simulink model "lookForPath_mod"  (Simulink 7.6)
settings: Solver=FixedStepDiscrete  StartTime=0.0  StopTime=0  RelTol=1e-3
values from neighbouring files (symbols this model uses):
  Track_HueHigher = .1    (= 0.1)    [VisionConstants.m]
  Track_HueLower = .25    (= 0.25)    [VisionConstants.m]
  Track_Min_Eccentricity = 0.9    [VisionConstants.m]
  Track_Saturation = 0.5    [VisionConstants.m]
undefined symbols (not defined in the file or in its folder): Rec, SDTV
libraries: simulink x3, vipstatistics x1, vipconversions x1, viptextngfix x1
settings Model: Creator=auvt  LastModifiedBy=Administrator  RecordCoverage=on  CovHTMLOptions=-aTS=1 -bRG=1 -bTC=1 -hTR=0 -nFC=0 -scm=1 -bcm=1 -xEv=0  CovModelRefEnable=all  CovExternalEMLEnable=on

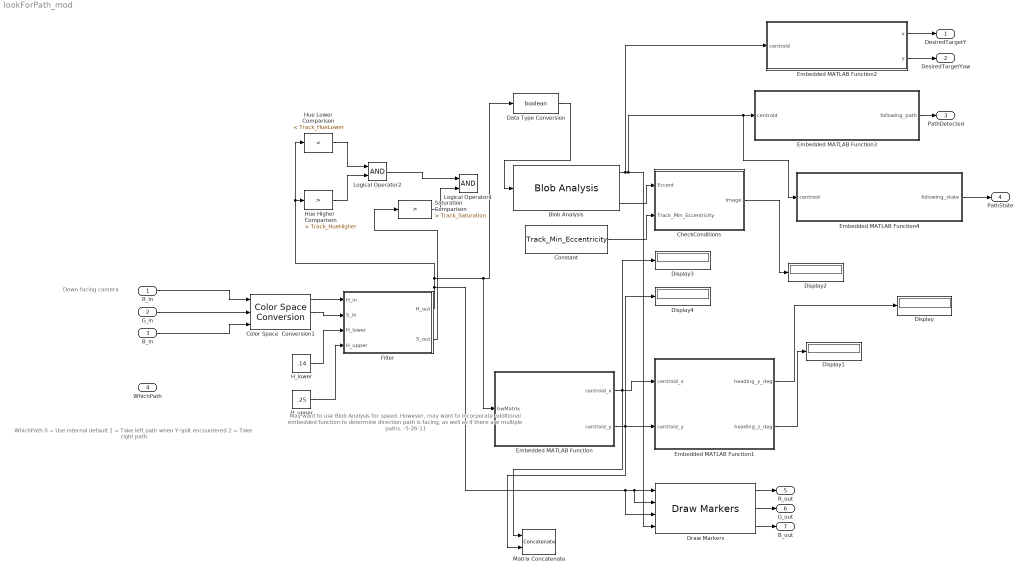
== system lookForPath_mod ==
  note: May want to use Blob Analysis for speed.
      | However, may want to incorporate
      | additional embedded function to
      | determine direction path is facing,
      | as well as if there are multiple paths.
      |
      | -5-26-11
  note: Down-facing camera
  note: WhichPath
      | 0 = Use internal default
      | 1 = Take left path when Y-split encountered
      | 2 = Take right path
  R_in : Inport  PortDimensions=[120 160]
  G_in : Inport  Port=2  PortDimensions=[120 160]
  B_in : Inport  Port=3  PortDimensions=[120 160]
  WhichPath : Inport  Port=4
  Blob Analysis : vipstatistics/Blob Analysis  Tag=vipblks_row_conv  DialogController=vipDDGCreate  DialogControllerArgs=DataTag0  area=off  centroid=on  bBox=on  majorAxis=off  minorAxis=off  angle=off  eccentricity=on  equivDiameterSq=off  extent=off  perimeter=off  maxBlobs=Max_Num_Blobs  warnIfNumBlobsExceeded=on  isCount=off  useMinArea=on  minArea=Min_Blob_Size  useMaxArea=on  maxArea=Max_Blob_Size  excludeBorderBlob=off  outDT=double  isOutVarDim=off  isFill=on  fillValues=-1  conn=8  isLabel=off  outputMode=Binary point scaling  outputWordLength=32  outputFracLength=16  firstCoeffMode=Binary point scaling  firstCoeffWordLength=16  firstCoeffFracLength=14  secondCoeffMode=Binary point scaling  secondCoeffWordLength=32  secondCoeffFracLength=16  accumMode=Binary point scaling  accumWordLength=32  accumFracLength=0  prodOutputMode=Binary point scaling  prodOutputWordLength=32  prodOutputFracLength=16  roundingMode=Floor  overflowMode=off
  CheckConditions : Stateflow chart  TreatAsAtomicUnit=on
  Color Space  Conversion1 : vipconversions/Color Space  Conversion  conversion=Obsolete  conversionActive=R'G'B' to HSV  wp_str=D65  rec=Rec. 601 (SDTV)  sys=1125/60/2:1  imagePorts=Separate color signals
  Constant : Constant  Value=Track_Min_Eccentricity  SampleTime=-1
  Data Type Conversion : DataTypeConversion  OutDataTypeStr=boolean
  Display{,1..4} (5 alike) : Display
  Draw Markers : viptextngfix/Draw Markers  DialogController=vipDDGCreate  DialogControllerArgs=DataTag1  shape=X-mark  size=7  fill=off  fillClrSource=Specify via dialog  display=User-specified value  intensity=200  color=[0 1 0]  opacity=0.6  viewport=Entire image  antialiasing=off  inType=Obsolete  imagePorts=Separate color signals  prodOutputMode=Binary point scaling  prodOutputWordLength=32  prodOutputFracLength=14  memoryMode=Specify word length  memoryWordLength=16  memoryFracLength=15  roundingMode=Floor  overflowMode=off
  Embedded MATLAB Function : Stateflow chart  TreatAsAtomicUnit=on
  Embedded MATLAB Function1 : Stateflow chart  TreatAsAtomicUnit=on
  Embedded MATLAB Function2 : Stateflow chart  TreatAsAtomicUnit=on
  Embedded MATLAB Function3 : Stateflow chart  TreatAsAtomicUnit=on
  Embedded MATLAB Function4 : Stateflow chart  TreatAsAtomicUnit=on
  Filter : Stateflow chart  TreatAsAtomicUnit=on
  H_lower : Constant  Value=.14  SampleTime=-1
  H_upper : Constant  Value=.25  SampleTime=-1
  Hue Higher Comparison : simulink/Logic and Bit Operations/Compare To Constant  SystemSampleTime=-1  relop=>  const=Track_HueHigher  LogicOutDataTypeMode=boolean  ZeroCross=off
  Hue Lower Comparison : simulink/Logic and Bit Operations/Compare To Constant  SystemSampleTime=-1  relop=<  const=Track_HueLower  LogicOutDataTypeMode=boolean  ZeroCross=off
  Logical Operator1 : Logic  AllPortsSameDT=off  OutDataTypeStr=boolean
  Logical Operator2 : Logic  AllPortsSameDT=off  OutDataTypeStr=boolean
  Matrix Concatenate : Concatenate  Mode=Multidimensional array  ConcatenateDimension=2
  Saturation Comparison : simulink/Logic and Bit Operations/Compare To Constant  SystemSampleTime=-1  relop=>  const=Track_Saturation  LogicOutDataTypeMode=boolean  ZeroCross=off
  DesiredTargetY : Outport  OutDataTypeStr=double
  DesiredTargetYaw : Outport  Port=2  OutDataTypeStr=double
  PathDetected : Outport  Port=3  OutDataTypeStr=double
  PathState : Outport  Port=4  OutDataTypeStr=double
  R_out : Outport  Port=5  OutDataTypeStr=double
  G_out : Outport  Port=6  OutDataTypeStr=double
  B_out : Outport  Port=7  OutDataTypeStr=double
  wires:
  CheckConditions/1(Image) -> Display2/1
  Constant/1 -> CheckConditions/2(Track_Min_Eccentricity)
  Saturation Comparison/1 -> Logical Operator1/2
  Logical Operator2/1 -> Logical Operator1/1
  Hue Higher Comparison/1 -> Logical Operator2/2
  Hue Lower Comparison/1 -> Logical Operator2/1
  Embedded MATLAB Function/1(centroid_x) -> Embedded MATLAB Function1/1(centroid_x), Display3/1, Matrix Concatenate/1
  Embedded MATLAB Function/2(centroid_y) -> Display4/1, Embedded MATLAB Function1/2(centroid_y), Matrix Concatenate/2
  Embedded MATLAB Function1/1(heading_y_deg) -> Display/1
  Embedded MATLAB Function1/2(heading_z_deg) -> Display1/1
  Blob Analysis/3 -> CheckConditions/1(Eccent)
  Blob Analysis/1 -> Embedded MATLAB Function2/1(centroid), Draw Markers/4, Embedded MATLAB Function3/1(centroid), Embedded MATLAB Function4/1(centroid)
  Embedded MATLAB Function2/2(y) -> DesiredTargetYaw/1
  Embedded MATLAB Function2/1(x) -> DesiredTargetY/1
  Embedded MATLAB Function3/1(following_path) -> PathDetected/1
  Embedded MATLAB Function4/1(following_state) -> PathState/1
  Filter/2(S_out) -> Saturation Comparison/1
  Filter/1(H_out) -> Draw Markers/1, Draw Markers/2, Draw Markers/3, Hue Lower Comparison/1, Hue Higher Comparison/1, Embedded MATLAB Function/1(bwMatrix), Data Type Conversion/1
  Color Space  Conversion1/1 -> Filter/1(H_in)
  Color Space  Conversion1/2 -> Filter/2(S_in)
  R_in/1 -> Color Space  Conversion1/1
  B_in/1 -> Color Space  Conversion1/3
  Draw Markers/1 -> R_out/1
  G_in/1 -> Color Space  Conversion1/2
  Draw Markers/2 -> G_out/1
  Draw Markers/3 -> B_out/1
  H_lower/1 -> Filter/3(H_lower)
  H_upper/1 -> Filter/4(H_upper)
  Data Type Conversion/1 -> Blob Analysis/1

== matlab function CheckConditions ==
  data: Eccent input double; Image output double; Track_Min_Eccentricity input double
function Image = CheckConditions(Eccent, Track_Min_Eccentricity)
% This function checks the conditions to decide if a track is present

if(Eccent > Track_Min_Eccentricity)
    Image = 1;
else
    Image = 0;
end

return

== matlab function Embedded MATLAB Function ==
  data: bwMatrix input double; centroid_x output double; centroid_y output double

function [centroid_x, centroid_y] = CentroidVertScan(bwMatrix)

centroid_x = 0;
centroid_y = 0;

%{
%Author: Yama Habib
%Revision: 10/27/2010
%CentroidVertScan takes a black and white matrix (the expected output of
%the blob detection algorithm) with a single (rectangular) object detected,
%and returns the raw matrix coordinate of the centroid of the object. To
%convert to an angular heading, use the Centroid2Heading function.

%Should these be parameters? I think they're fine as constants.
WIDTH = size(bwMatrix, 2);
HEIGHT = size(bwMatrix, 1);

%increase the x step to increase efficiency. The further this
%number is from 1, the closer the object will have to be to be detected
%NOTE: find the max distance the hedge will be from the AUV, then find the
%optimal (lowest working) x step for that distance!
X_STEP = 1;
Y_STEP = 1;

%Don't detect lines unless they are longer than HEIGHT*THRESHOLD
THRESHOLD = 0.1;

%Allocate arrays...allocate more or less memory depending on how many lines
%are found in the average case
lineLengths = zeros(WIDTH,1);
lineMidpts_y = zeros(WIDTH,1);
lineMidpts_x = zeros(WIDTH,1);

%Find vertical lines
index = 1;
i = 1;
while(i <= WIDTH)
    j = 1;
    while(j <= HEIGHT)
        %skip whitespace
        while(bwMatrix(j,floor(i)) == 0)
%        while(bwMatrix(floor(i),j) == 0)
            j = j+1;
            if(j > HEIGHT)
                break;
            end
        end
        %count contiguous blackspace
        if(j <= HEIGHT)
            length = 0;
            midpt = j;
            while(bwMatrix(floor(i),j) ~= 0)
                length = length+1;
                j = j+1;
                if(j > HEIGHT)
                    break;
                end
            end
            midpt = midpt + length/2;
            %only register as a line if longer than HEIGHT*THRESHOLD
            if(length > HEIGHT*THRESHOLD)
                lineLengths(index) = length;
                lineMidpts_y(index) = midpt;
                lineMidpts_x(index) = floor(i);
                index = index+1;
            end
        end
        %rinse, repeat
    end
    i = i+X_STEP;
end

%Find maximum (longest rightmost) and minimum (longest leftmost) vertical
%lines
i = 1;
min = 1;
max = 1;
while(i <= index);
    
    % The following comparisons seek to minimize and maximize the metric
    %   " length*( width - x_midpt ) ". This effectively finds the largest
    %   leftmost and rightmost vertical lines.
    
    % This if statement should be "<" instead of ">" ??
    if(lineLengths(i)*(WIDTH-lineMidpts_x(i)) > lineLengths(min)*(WIDTH-lineMidpts_x(min)))
        min = i;
    end
    % This if statement should be correct
    if(lineLengths(i)*(lineMidpts_x(i)) >= lineLengths(max)*(lineMidpts_x(max)))
        max = i;
    end
    i = i+1;
end

%The centroid is (should be) the midpoint between the max's midpoint and
%the min's midpoint
% The assumption made is that the rightmost and leftmost lines bound a
% vertically-oriented rectangular path
centroid_x = (lineMidpts_x(min) + lineMidpts_x(max))/2;
centroid_y = (lineMidpts_y(min) + lineMidpts_y(max))/2;
end











%}










%{

% The following is the old code:







function [centroid_x, centroid_y] = CentroidVertScan(bwMatrix)
%Author: Yama Habib
%Revision: 10/27/2010
%CentroidVertScan takes a black and white matrix (the expected output of
%the blob detection algorithm) with a single (rectangular) object detected,
%and returns the raw matrix coordinate of the centroid of the object. To
%convert to an angular heading, use the Centroid2Heading function.

%Should these be parameters? I think they're fine as constants.
WIDTH = size(bwMatrix, 2);
HEIGHT = size(bwMatrix, 1);
%WIDTH = 160;
%HEIGHT = 120;

%increase the x step to increase efficiency. The further this
%number is from 1, the closer the object will have to be to be detected
%NOTE: find the max distance the hedge will be from the AUV, then find the
%optimal (lowest working) x step for that distance!
X_STEP = 1;

%Don't detect lines unless they are longer than HEIGHT*THRESHOLD
THRESHOLD = 0.1;

%Allocate arrays...allocate more or less memory depending on how many lines
%are found in the average case
lineLengths = zeros(WIDTH,1);
lineMidpts_y = zeros(WIDTH,1);
lineMidpts_x = zeros(WIDTH,1);

%Find vertical lines
index = 1;
i = 1;
while(i <= WIDTH)
    j = 1;
    while(j <= HEIGHT)
        %skip whitespace
        while(bwMatrix(j,floor(i)) == 0)
%        while(bwMatrix(floor(i),j) == 0)
            j = j+1;
            if(j > HEIGHT)
                break;
            end
        end
        %count contiguous blackspace
        if(j <= HEIGHT)
            length = 0;
            midpt = j;
            while(bwMatrix(floor(i),j) ~= 0)
                length = length+1;
                j = j+1;
                if(j > HEIGHT)
                    break;
                end
            end
            midpt = midpt + length/2;
            %only register as a line if longer than HEIGHT*THRESHOLD
            if(length > HEIGHT*THRESHOLD)
                lineLengths(index) = length;
                lineMidpts_y(index) = midpt;
                lineMidpts_x(index) = floor(i);
                index = index+1;
            end
        end
        %rinse, repeat
    end
    i = i+X_STEP;
end

%Find maximum (longest rightmost) and minimum (longest leftmost) vertical
%lines
i = 1;
min = 1;
max = 1;
while(i <= index);
    
    % The following comparisons seek to minimize and maximize the metric
    %   " length*( width - x_midpt ) ". This effectively finds the largest
    %   leftmost and rightmost vertical lines.
    
    % This if statement should be "<" instead of ">" ??
    if(lineLengths(i)*(WIDTH-lineMidpts_x(i)) > lineLengths(min)*(WIDTH-lineMidpts_x(min)))
        min = i;
    end
    % This if statement should be correct
    if(lineLengths(i)*(lineMidpts_x(i)) >= lineLengths(max)*(lineMidpts_x(max)))
        max = i;
    end
    i = i+1;
end

%The centroid is (should be) the midpoint between the max's midpoint and
%the min's midpoint
% The assumption made is that the rightmost and leftmost lines bound a
% vertically-oriented rectangular path
centroid_x = (lineMidpts_x(min) + lineMidpts_x(max))/2;
centroid_y = (lineMidpts_y(min) + lineMidpts_y(max))/2;
end

%}

== matlab function Embedded MATLAB Function1 ==
  data: centroid_x input double; heading_y_deg output double; centroid_y input double; heading_z_deg output double
function [heading_y_deg, heading_z_deg] = Centroid2Heading(centroid_x, centroid_y)
%Author: Yama Habib
%Revision: 10/27/2010
%Centroid2Heading takes a raw matrix centroid coordinate and converts
%it into a correction heading, in degrees (i.e. heading_y_deg = -30,
%heading_z_deg = 45 means that in order to orient yourself so that the
%object in question is centered in the video feed, you need to turn 30
%degrees to the left and 45 degrees upwards, assuming the camera is mounted
%on the front) The probability that this function will return exactly 0
%degrees is laughably low, so applying a reasonable threshold to the
%result is strongly recommended.

%Should these be parameters? I think they're fine as constants.
WIDTH = 160;
HEIGHT = 120;
MAXANGLE = 130;

heading_y_deg = ((centroid_x-(WIDTH/2)) / (WIDTH/2)) * (MAXANGLE/2);
heading_z_deg = ((centroid_y-(HEIGHT/2)) / (HEIGHT/2)) * (MAXANGLE/2);
end

== matlab function Embedded MATLAB Function2 ==
  data: x output double; centroid input double; y output double
function [x, y] = separate_centroids(centroid)

x = centroid(1);
y = centroid(2);

== matlab function Embedded MATLAB Function3 ==
  data: following_path output double; centroid input double
function following_path = separate_centroids(centroid)

% If at least one path element is found, then report that the path is being
% followed
if(size(centroid,1) ~= 0)
    following_path = 1;
else
    following_path = 0;
end

== matlab function Embedded MATLAB Function4 ==
  data: following_state output double; centroid input double
function following_state = separate_centroids(centroid)

% Editing note:
%   -centroid is not a useful input. This function has yet to be written.
%      -5-27-11


% Determine whether:
%   0 = No path is being followed
%   1 = A single path (can be made up of n path elements along one line)
%         is being followed
%   2 = A Y-split is being encountered
%   3 = A Y-join is being encountered

following_state = 1;

== matlab function Filter ==
  data: H_in input double; S_in input double; H_lower input double; H_upper input double; H_out output double; S_out output double
function [H_out, S_out] = path_filter(H_in, S_in, H_lower, H_upper)
% This function extracts the pixels containing hues that path elements are
%   expected to have


% Initialize
H_out = double(H_in);
S_out = double(S_in);


% Set values outside valid ranges to zero
for i = 1:size(H_in,1)
    for j = 1:size(H_in,2)
        
        if( H_in(i,j) >= H_lower && H_in(i,j) <= H_upper )
            H_out(i,j) = 1;
        else
            H_out(i,j) = 0;
        end
        
    end
end



return
